simulink model "Sub3_2023"  (R2023b)
settings: Solver=FixedStepDiscrete  StartTime=0.0  StopTime=4.5  FixedStep=75e-6  RelTol=1e-3  EnableMultiTasking=on
undefined symbols (not defined in the file or in its folder): D1, D11, Delta
libraries: spsSeriesRLCBranchLib x41, spsLoadFlowBusLib x29, spsDistributedParametersLineLib x19, spsThreePhaseSeriesRLCLoadLib x15, spsThreePhaseTransformerTwoWindingsLib x13, spsThreePhaseParallelRLCLoadLib x11, spsThreePhaseVIMeasurementLib x11, spsSynchronousMachinepuStandardLib x7, spsExcitationSystemLib x7, spsHydraulicTurbineandGovernorLib x7, spsGenericPowerSystemStabilizerLib x7, spsMultiBandPowerSystemStabilizerLib x7
(part 3 of 5)

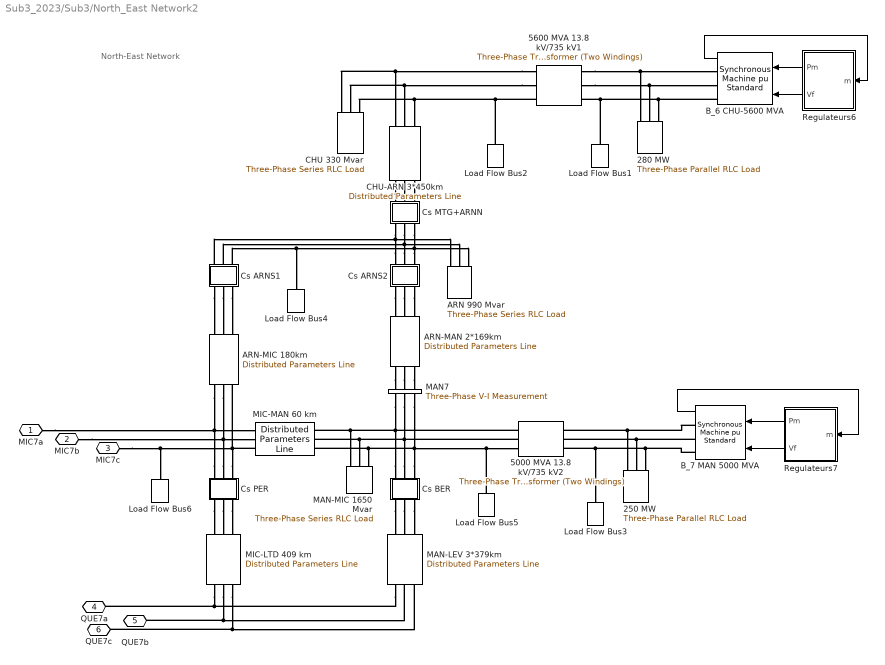
== system Sub3_2023/Sub3/North_East Network2 ==
  note: North-East Network
  250 MW : spsThreePhaseParallelRLCLoadLib/Three-Phase Parallel RLC Load  LConnTagsString=A|B|C  Configuration=Y (grounded)  NominalVoltage=(13800)*1  Vabc=[1e3 1e3 1e3]  Vabcp=[1e3 1e3 1e3]  NominalFrequency=60  UnbalancedPower=off  ActivePower=250000000  InductivePower=0  CapacitivePower=0  Pabc=[10e3 9e3 11e3]  QLabc=[100 90 110]  QCabc=[100 90 110]  Pabcp=[10e3 9e3 11e3]  QLabcp=[100 90 110]  QCabcp=[100 90 110]  Measurements=None  LoadType=constant PQ
  280 MW : spsThreePhaseParallelRLCLoadLib/Three-Phase Parallel RLC Load  LConnTagsString=A|B|C  Configuration=Y (grounded)  NominalVoltage=(13800)*1  Vabc=[1e3 1e3 1e3]  Vabcp=[1e3 1e3 1e3]  NominalFrequency=60  UnbalancedPower=off  ActivePower=280000000  InductivePower=0  CapacitivePower=0  Pabc=[10e3 9e3 11e3]  QLabc=[100 90 110]  QCabc=[100 90 110]  Pabcp=[10e3 9e3 11e3]  QLabcp=[100 90 110]  QCabcp=[100 90 110]  Measurements=None  LoadType=constant PQ
  5000 MVA 13.8 kV/735 kV2 : spsThreePhaseTransformerTwoWindingsLib/Three-Phase Transformer (Two Windings)  Winding1Connection=Delta (D1)  Winding2Connection=Yg  CoreType=Three single-phase transformers  SetSaturation=off  Hysteresis=off  DataFile='basic_model'  SetInitialFlux=off  Measurements=None  UNITS=pu  NominalPower=[ 5000e6 60 ]  Winding1="[ 13.8e3 0.002  0.0]"  Winding2=[ 735e3 0.002 0.12]  Rm=500  Lm=500  L0=0.5  Saturation="[ 0,0  ;  0.005,1.2  ;  1.0,1.4 ]"  InitialFluxes=[ 0.8 , -0.8 , 0.7 ]  BreakLoop=off  DiscreteSolver=Trapezoidal iterative  DataType=off  TransfoNumber=0
  5600 MVA 13.8 kV/735 kV1 : spsThreePhaseTransformerTwoWindingsLib/Three-Phase Transformer (Two Windings)  Winding1Connection=Delta (D1)  Winding2Connection=Yg  CoreType=Three single-phase transformers  SetSaturation=off  Hysteresis=off  DataFile='basic_model'  SetInitialFlux=off  Measurements=None  UNITS=pu  NominalPower=[ 5600e6 60 ]  Winding1="[ 13.8e3 0.002  0.0]"  Winding2=[ 735e3 0.002 0.12]  Rm=500  Lm=500  L0=0.5  Saturation="[ 0,0  ;  0.005,1.2  ;  1.0,1.4 ]"  InitialFluxes=[ 0.8 , -0.8 , 0.7 ]  BreakLoop=off  DiscreteSolver=Trapezoidal iterative  DataType=off  TransfoNumber=0
  ARN 990 Mvar : spsThreePhaseSeriesRLCLoadLib/Three-Phase Series RLC Load  LConnTagsString=A|B|C  Configuration=Y (grounded)  NominalVoltage=735e3  Vabc=[1e3 1e3 1e3]  Vabcp=[1e3 1e3 1e3]  NominalFrequency=60  UnbalancedPower=off  ActivePower=3300000  InductivePower=990e6  CapacitivePower=0  Pabc=[10e3 9e3 11e3]  QLabc=[100 90 110]  QCabc=[100 90 110]  Pabcp=[10e3 9e3 11e3]  QLabcp=[100 90 110]  QCabcp=[100 90 110]  Measurements=None  LoadType=constant Z
  ARN-MAN 2*169km : spsDistributedParametersLineLib/Distributed Parameters Line  Phases=3  Length=169  Frequency=60  Resistance="[0.01273  0.3864]/2"  Inductance="[0.9337e-3  4.1264e-3]/2"  Capacitance=[12.74e-9 7.751e-9]*2  x1=[-0.000975 1.67472397753016e-09 276427.2961151 -784420.047795512;-0.0009 1.60147333737436e-09 298492.841238193 -776291.834335293;-0.000825 1.52694250393602e-09 320319.775751095 -767543.06506037;-0.00075 1.45119105602304e-09 341890.651536318 -758180.733603041;-0.000675 1.37427954818385e-09 363188.225165806 -748212.324067824;-0.0006 1.29626946230102e-09 384195.471685062 -737645.805048779;-0.000525 1.21722315844361e-09 404895.598222641 -726489.623259537;-0.00045 1.13720382501748e-09 425272.057414111 -714752.696781126;-0.000375 1.05627542825344e-09 445308.560629765 -702444.407932991;-0.0003 9.74502661073603e-10 464989.090995501 -689574.595772914;-0.000225 8.91950891376898e-10 484297.916196467 -676153.548231822;-0.00015 8.08686109784932e-10 503219.601053231 -662191.993889769;-7.5e-05 7.24774876890116e-10 521739.019860433 -647701.093399678]  x2=[-0.000975 1.45072483719961e-09 170603.864508841 -782532.609847126;-0.0009 1.40774718437802e-09 192658.333570929 -777396.800423857;-0.000825 1.36364419999649e-09 214558.794508932 -771639.551892899;-0.00075 1.31845113930594e-09 236287.740429464 -765265.466510639;-0.000675 1.2722041289476e-09 257827.80154562 -758279.639623405;-0.0006 1.22494013807397e-09 279161.759062119 -750687.655594323;-0.000525 1.17669694879617e-09 300272.558939742 -742495.583339266;-0.00045 1.12751312598156e-09 321143.325528072 -733709.97147545;-0.000375 1.07742798642558e-09 341757.375055633 -724337.843086576;-0.0003 1.02648156742245e-09 362098.228966637 -714386.690108679;-0.000225 9.7471459476002e-10 382149.627093695 -703864.467341192;-0.00015 9.2216845016417e-10 401895.540655938 -692779.586088001;-7.5e-05 8.68885138218909e-10 421320.18507219 -681140.907433573]  x3=[-0.000975 -1.05058696200227e-12 1329.17201367209 -2414.87241463344;-0.0009 -1.27237442727808e-12 1396.90953145506 -2376.33167069217;-0.000825 -1.4931447759047e-12 1463.53038113202 -2335.89132357245;-0.00075 -1.71272152744335e-12 1528.98130701506 -2293.58370066899;-0.000675 -1.93092915559848e-12 1593.20998863548 -2249.44262204823;-0.0006 -2.14759322853083e-12 1656.16508256791 -2203.50337341303;-0.000525 -2.36254054829557e-12 1717.79626347352 -2155.80267789586;-0.00045 -2.57559928929408e-12 1778.05426432926 -2106.37866670286;-0.000375 -2.78659913562873e-12 1836.89091581125 -2055.27084863238;-0.0003 -2.99537141725075e-12 1894.2591848005 -2002.52007849219;-0.000225 -3.20174924479254e-12 1950.11321198057 -1948.16852444085;-0.00015 -3.40556764297644e-12 2004.40834849671 -1892.25963427904;-7.5e-05 -3.60666368249349e-12 2057.10119164754 -1834.83810071814]  x4=[-0.000975 1.05706410418254e-11 681.724417840617 -9455.17189861369;-0.0009 1.03719190093797e-11 948.756484621806 -9432.11979189245;-0.000825 1.01649058235736e-11 1215.03012998565 -9401.52779292584;-0.00075 9.94976696758033e-12 1480.33249885417 -9363.42035648977;-0.000675 9.72667442010975e-12 1744.45151257295 -9317.82794508585;-0.0006 9.49580651793084e-12 2007.17603844358 -9264.78700459018;-0.000525 9.25734781331221e-12 2268.2960584999 -9204.33993511903;-0.00045 9.01148892649379e-12 2527.60283739316 -9136.53505713488;-0.000375 8.75842639330793e-12 2784.88908925182 -9061.42657281972;-0.0003 8.49836250807169e-12 3039.94914338276 -8979.07452274673;-0.000225 8.23150516187579e-12 3292.57910868127 -8889.5447378847;-0.00015 7.95806767639975e-12 3542.57703661844 -8792.9087869738;-7.5e-05 7.67826863338571e-12 3789.74308267579 -8689.24391931461]  x5=0.000955765248222805  V1=ones(3,3)  V2=ones(3,3)  I1=ones(3,3)  I2=ones(3,3)  nHarmo=1  Measurements=None  Decoupling=on  VsMag0=[679080.965035231 679082.342856258 679080.506296754]  VrMag0=[653943.402704874 653944.061381525 653943.21471976]  VsAngle0=[10.4723030523858 -109.527808757282 130.47214647176]  VrAngle0=[3.35889302260881 -116.641159315006 123.358816875026]  IsMag0=[2259.59659727673 2259.62910082009 2259.62302792986]  IrMag0=[7771.0084515065 7771.00049259901 7770.97273571619]  IsAngle0=[19.8888438810525 -100.110858095203 139.888279140942]  IrAngle0=[-4.81594167232723 -124.81621186364 115.183974051697]
      settings: AttributesFormatString=\n  LibrarySourceBlock=sps_lib/Power Grid Elements/Distributed Parameters Line
  ARN-MIC 180km : spsDistributedParametersLineLib/Distributed Parameters Line  Phases=3  Length=180  Frequency=60  Resistance="[0.01273  0.3864]"  Inductance="[0.9337e-3  4.1264e-3]"  Capacitance=[12.74e-9 7.751e-9]  x1=[-0.00105 1.24724783260845e-09 262529.955827382 -774207.772445515;-0.000975 1.17944476350714e-09 284312.349574646 -766476.523484134;-0.0009 1.110698864308e-09 305867.468379784 -758132.564917363;-0.000825 1.04106508943099e-09 327178.081410629 -749182.566778015;-0.00075 9.70599103050325e-10 348227.153289186 -739633.683557663;-0.000675 8.99357234597342e-10 368997.857709458 -729493.548487449;-0.0006 8.27396433731648e-10 389473.590888134 -718770.2674362;-0.000525 7.5477422481642e-10 409637.9848374 -707472.412430716;-0.00045 6.81548660934306e-10 429474.920449258 -695609.014803426;-0.000375 6.07778277480686e-10 448968.540380895 -683189.557972877;-0.0003 5.33522045371367e-10 468103.261730801 -670223.969862836;-0.000225 4.58839323902139e-10 486863.7884955 -656722.614966056;-0.00015 3.83789813297861e-10 505235.12379694 -642696.286059066;-7.5e-05 3.08433506989013e-10 523202.581870775 -628156.195574583]  x2=[-0.00105 4.58025582629427e-09 126759.491965629 -811882.989724212;-0.000975 4.52463715432621e-09 149661.239004177 -807974.954382897;-0.0009 4.46540155664625e-09 172443.34913816 -803421.036225481;-0.000825 4.40259638528484e-09 195087.610697313 -798224.87558446;-0.00075 4.33627184573503e-09 217575.922205416 -792390.626191147;-0.000675 4.26648095681891e-09 239890.30685033 -785922.95185524;-0.0006 4.19327950830526e-09 262012.926854394 -778827.022736644;-0.000525 4.116726016312e-09 283926.097733662 -771108.511212526;-0.00045 4.03688167652932e-09 305612.302434616 -762773.5873429;-0.000375 3.95381031530078e-09 327054.20533703 -753828.913938379;-0.0003 3.86757833860152e-09 348234.666111794 -744281.641234026;-0.000225 3.77825467895431e-09 369136.753422638 -734139.401173561;-0.00015 3.68591074032598e-09 389743.758460777 -723410.301308507;-7.5e-05 3.59062034104816e-09 410039.208301682 -712102.918317136]  x3=[-0.00105 2.96537177276768e-12 -44.8517351582774 -825.879343626536;-0.000975 3.21260661019266e-12 -21.4861584035534 -826.817643960417;-0.0009 3.45727333904798e-12 1.89659405744908 -827.094998920449;-0.000825 3.69917637649412e-12 25.2778304101809 -826.711186793323;-0.00075 3.93812234894418e-12 48.6388600520466 -825.66651439258;-0.000675 4.17392024664379e-12 71.9610085333863 -823.961816813352;-0.0006 4.40638157636136e-12 95.2256324855447 -821.598456764802;-0.000525 4.63532051206668e-12 118.414134524095 -818.578323480792;-0.00045 4.86055404347744e-12 141.507978115304 -814.90383120966;-0.000375 5.08190212235481e-12 164.488702393952 -810.577917284306;-0.0003 5.29918780643128e-12 187.337936920669 -805.604039774133;-0.000225 5.51223740085559e-12 210.037416366977 -799.98617472072;-0.00015 5.7208805970417e-12 232.568995116322 -793.728812959434;-7.5e-05 5.92495060881096e-12 254.914661769395 -786.836956529526]  x4=[-0.00105 4.18543085449922e-12 787.856966725132 -5164.02437043793;-0.000975 3.74166953826904e-12 933.532622338205 -5139.68710729476;-0.0009 3.29491718865944e-12 1078.46202625651 -5111.24125691787;-0.000825 2.84553093266314e-12 1222.52932413205 -5078.7095584848;-0.00075 2.39387000277736e-12 1365.6193507712 -5042.11801733755;-0.000675 1.94029544983879e-12 1507.61772219602 -5001.49588419424;-0.0006 1.48516985440514e-12 1648.41092708104 -4956.87563176655;-0.000525 1.02885703691374e-12 1787.88641749249 -4908.29292880156;-0.00045 5.71721766849072e-13 1925.93269885737 -4855.78661156869;-0.000375 1.1412947115162e-13 2062.43941909055 -4799.39865281457;-0.0003 -3.43554057898831e-13 2197.29745680848 -4739.17412821064;-0.000225 -8.00962955091952e-13 2330.39900855922 -4675.16118032042;-0.00015 -1.25773157475392e-12 2461.63767499882 -4607.41098011501;-7.5e-05 -1.71349478303896e-12 2590.90854594535 -4535.97768606785]  x5=0.00101797482059234  V1=ones(3,3)  V2=ones(3,3)  I1=ones(3,3)  I2=ones(3,3)  nHarmo=1  Measurements=None  Decoupling=on  VsMag0=[667492.500318924 667493.817536521 667492.030186015]  VrMag0=[670930.718084371 670931.402748966 670930.538861449]  VsAngle0=[11.411536339946 -108.588575536847 131.411382483005]  VrAngle0=[1.55396261636306 -118.446088813405 121.553886266144]  IsMag0=[678.171382863083 678.181184846405 678.186053011925]  IrMag0=[4283.30300695141 4283.29854095568 4283.28683546869]  IsAngle0=[-10.4293295371495 -130.428376510203 109.570429815951]  IrAngle0=[1.35460954054908 -118.645605751909 121.354553630563]
      settings: AttributesFormatString=\n  LibrarySourceBlock=sps_lib/Power Grid Elements/Distributed Parameters Line
  "B_6 CHU-5600 MVA " : spsSynchronousMachinepuStandardLib/Synchronous Machine pu Standard  PresetModel=No  MechanicalLoad=Mechanical power Pm  ShowDetailedParameters=on  RotorType=Salient-pole  Units=per unit standard parameters  MeasurementBus=off  NominalParameters="[ 5600E6  13800   60 ]"  Reactances1=[ 31 32 33 34 35 36 37 ]  Reactances2=[ 1.305, 0.296, 0.252, 0.474, 0.243, 0.18 ]  dAxisTimeConstants=Short-circuit  qAxisTimeConstants=Open-circuit  TimeConstants1=[]  TimeConstants2=[]  TimeConstants3=[]  TimeConstants4=[]  TimeConstants5=[ 1.01, 0.053, 0.1 ]  TimeConstants6=[]  TimeConstants7=[]  TimeConstants8=[]  StatorResistance=2.8544e-3  Mechanical="[ 4.0 0  32]"  PolePairs=32  InitialConditions=[0 -61.7964 0.894782 0.894782 0.894782 8.48442 -111.516 128.484 1.31361]  SetSaturation=off  Saturation=[0.6404,0.7127,0.8441,0.9214,0.9956,1.082,1.19,1.316,1.457;0.7,0.7698,0.8872,0.9466,0.9969,1.046,1.1,1.151,1.201]  LoadFlowParameters=[1 5000000000 0 0 0]  TsPowergui=0  TsBlock=-1  IterativeModel=Trapezoidal non iterative  IterativeDiscreteModel=Trapezoidal non iterative  BusType=PV  Pref=5000000000  Qref=0  Qmin=-Inf  Qmax=Inf  PLF=0  QLF=0
  B_7 MAN 5000 MVA : spsSynchronousMachinepuStandardLib/Synchronous Machine pu Standard  PresetModel=No  MechanicalLoad=Mechanical power Pm  ShowDetailedParameters=on  RotorType=Salient-pole  Units=per unit standard parameters  MeasurementBus=off  NominalParameters="[ 5000E6  13800   60 ]"  Reactances1=[ 31 32 33 34 35 36 37 ]  Reactances2=[ 1.305, 0.296, 0.252, 0.474, 0.243, 0.18 ]  dAxisTimeConstants=Short-circuit  qAxisTimeConstants=Open-circuit  TimeConstants1=[]  TimeConstants2=[]  TimeConstants3=[]  TimeConstants4=[]  TimeConstants5=[ 1.01, 0.053, 0.1 ]  TimeConstants6=[]  TimeConstants7=[]  TimeConstants8=[]  StatorResistance=2.8544e-3  Mechanical="[ 3.7 0  32]"  PolePairs=32  InitialConditions=[0 -81.9543 0.907703 0.907703 0.907703 -8.76021 -128.76 111.24 1.25655]  SetSaturation=off  Saturation=[0.6404,0.7127,0.8441,0.9214,0.9956,1.082,1.19,1.316,1.457;0.7,0.7698,0.8872,0.9466,0.9969,1.046,1.1,1.151,1.201]  LoadFlowParameters=[1 4500000000 0 0 0]  TsPowergui=0  TsBlock=-1  IterativeModel=Trapezoidal non iterative  IterativeDiscreteModel=Trapezoidal non iterative  BusType=PV  Pref=4500000000  Qref=0  Qmin=-Inf  Qmax=Inf  PLF=0  QLF=0
  CHU 330 Mvar : spsThreePhaseSeriesRLCLoadLib/Three-Phase Series RLC Load  LConnTagsString=A|B|C  Configuration=Y (grounded)  NominalVoltage=735e3  Vabc=[1e3 1e3 1e3]  Vabcp=[1e3 1e3 1e3]  NominalFrequency=60  UnbalancedPower=off  ActivePower=1100000  InductivePower=330e6  CapacitivePower=0  Pabc=[10e3 9e3 11e3]  QLabc=[100 90 110]  QCabc=[100 90 110]  Pabcp=[10e3 9e3 11e3]  QLabcp=[100 90 110]  QCabcp=[100 90 110]  Measurements=None  LoadType=constant Z
  CHU-ARN 3*450km : spsDistributedParametersLineLib/Distributed Parameters Line  Phases=3  Length=450  Frequency=60  Resistance="[0.01273  0.3864]/3"  Inductance="[0.9337e-3  4.1264e-3]/3"  Capacitance=[12.74e-9 7.751e-9]*3  x1=[-0.00255 1.77535384487348e-09 0 0;-0.002475 1.68842898528115e-09 0 0;-0.0024 1.60015442139181e-09 0 0;-0.002325 1.5106007185412e-09 0 0;-0.00225 1.41983946458915e-09 0 0;-0.002175 1.32794321269338e-09 0 0;-0.0021 1.23498542331159e-09 0 0;-0.002025 1.14104040547832e-09 0 0;-0.00195 1.04618325740342e-09 0 0;-0.001875 9.50489806439687e-10 0 0;-0.0018 8.54036548467669e-10 0 0;-0.001725 7.56900586746003e-10 0 0;-0.00165 6.59159570276259e-10 0 0;-0.001575 5.60891631731516e-10 242668.421457002 -732167.508894334;-0.0015 4.62175324998297e-10 263270.288908672 -725014.59046711;-0.001425 3.63089562381793e-10 283661.702119559 -717282.106469362;-0.00135 2.63713551524579e-10 303826.360505941 -708976.238130487;-0.001275 1.64126732089228e-10 323748.144748434 -700103.62503455;-0.0012 6.44087122554682e-11 343411.129677528 -690671.359812705;-0.001125 -3.53607949173821e-11 362799.597003924 -680686.982473452;-0.00105 -1.35102035211814e-10 381898.047883495 -670158.47437527;-0.000975 -2.34735277006428e-10 400691.215306824 -659094.251846441;-0.0009 -3.34180875012173e-10 419164.076303418 -647503.159457166;-0.000825 -4.33359333939572e-10 437301.86395084 -635394.462949351;-0.00075 -5.3219137204604e-10 455090.079179163 -622777.841829716;-0.000675 -6.30597984512496e-10 472514.502361302 -609663.381632143;-0.0006 -7.28500506598605e-10 489561.204679968 -596061.565855456;-0.000525 -8.2582067652617e-10 506216.55926215 -581983.267583072;-0.00045 -9.22480698040401e-10 522467.252072231 -567439.740791224;-0.000375 -1.01840330259905e-09 538300.292555022 -552442.611352707;-0.0003 -1.11351181113969e-09 553703.024020216 -537003.86774333;-0.000225 -1.2077301953758e-09 568663.133759948 -521135.851458514;-0.00015 -1.30098313857263e-09 583168.66289139 -504851.247147688;-7.5e-05 -1.39319609575419e-09 597208.015916497 -488163.072474375]  x2=[-0.00255 2.72407888436873e-09 0 0;-0.002475 2.6953160484316e-09 0 0;-0.0024 2.66439861808508e-09 0 0;-0.002325 2.63135130824993e-09 0 0;-0.00225 2.59620053643998e-09 0 0;-0.002175 2.55897440164441e-09 0 0;-0.0021 2.51970266186578e-09 0 0;-0.002025 2.478416710332e-09 0 0;-0.00195 2.43514955040103e-09 0 0;-0.001875 2.38993576917851e-09 0 0;-0.0018 2.34281150986935e-09 0 0;-0.001725 2.29381444288541e-09 0 0;-0.00165 2.24298373573238e-09 0 0;-0.001575 2.1903600216998e-09 -54170.2857367538 -807523.190587141;-0.0015 2.1359853673795e-09 -31319.4766466804 -808731.868853748;-0.001425 2.0799032390382e-09 -8443.63124617975 -809294.059238405;-0.00135 2.02215846787119e-09 14438.9638639472 -809209.312334721;-0.001275 1.96279721416503e-09 37310.0166872849 -808477.695888074;-0.0012 1.90186693039767e-09 60151.2444541452 -807099.794741458;-0.001125 1.83941632330569e-09 82944.3882365337 -805076.710367967;-0.00105 1.77549531494887e-09 105671.227544058 -802410.059990295;-0.000975 1.71015500280328e-09 128313.594889107 -799101.975287951;-0.0009 1.64344761891469e-09 150853.390309666 -795155.100693233;-0.000825 1.57542648814513e-09 173272.595838145 -790572.591277302;-0.00075 1.50614598554578e-09 195553.289904671 -785358.110228069;-0.000675 1.43566149289039e-09 217677.661663313 -779515.825921903;-0.0006 1.36402935440395e-09 239628.025229801 -773050.408591487;-0.000525 1.29130683172194e-09 261386.833819352 -765967.02659251;-0.00045 1.21755205811631e-09 282936.693773301 -758271.342272164;-0.000375 1.1428239920246e-09 304260.378463324 -749969.507442746;-0.0003 1.06718236991945e-09 325340.842062143 -741068.158463997;-0.000225 9.90687658556226e-10 346161.2331697 -731574.410938095;-0.00015 9.13401006636783e-10 366704.908283905 -721495.854021552;-7.5e-05 8.35384195928139e-10 386955.445105201 -710840.544358562]  x3=[-0.00255 5.00391490531751e-12 0 0;-0.002475 4.937944497013e-12 0 0;-0.0024 4.86802677143067e-12 0 0;-0.002325 4.79421761973056e-12 0 0;-0.00225 4.71657604381923e-12 0 0;-0.002175 4.6351641091845e-12 0 0;-0.0021 4.55004689528128e-12 0 0;-0.002025 4.46129244350803e-12 0 0;-0.00195 4.36897170281549e-12 0 0;-0.001875 4.27315847299124e-12 0 0;-0.0018 4.17392934566519e-12 0 0;-0.001725 4.07136364308348e-12 0 0;-0.00165 3.96554335469944e-12 0 0;-0.001575 3.8565530716325e-12 -1464.09976005058 -2947.40439174839;-0.0015 3.74447991904734e-12 -1380.19037065337 -2987.6190390229;-0.001425 3.62941348650736e-12 -1295.17767819147 -3025.44542934972;-0.00135 3.51144575635815e-12 -1209.12964051052 -3060.85332489118;-0.001275 3.39067103019823e-12 -1122.11504309524 -3093.81442111735;-0.0012 3.26718585349578e-12 -1034.20344408345 -3124.30236943223;-0.001125 3.14108893841166e-12 -945.465118662299 -3152.29279823642;-0.00105 3.01248108489045e-12 -855.971002891393 -3177.76333240939;-0.000975 2.88146510008248e-12 -765.792636997571 -3200.69361119584;-0.0009 2.7481457161614e-12 -675.002108186754 -3221.06530448176;-0.000825 2.61262950660287e-12 -583.671993018531 -3238.86212744722;-0.00075 2.47502480099132e-12 -491.875299389569 -3254.06985358426;-0.000675 2.33544159842301e-12 -399.68540817222 -3266.67632606928;-0.0006 2.19399147957438e-12 -307.176014554971 -3276.67146748106;-0.000525 2.05078751750617e-12 -214.421069131637 -3284.0472878565;-0.00045 1.90594418727457e-12 -121.49471878639 -3288.79789107763;-0.000375 1.75957727442158e-12 -28.4712474218783 -3290.91947958492;-0.0003 1.61180378241786e-12 64.5749834221983 -3290.410357413;-0.000225 1.4627418391319e-12 157.569594012558 -3287.27093154632;-0.00015 1.31251060240043e-12 250.438245880359 -3281.5037115939;-7.5e-05 1.1612301647755e-12 343.106701246237 -3273.11330778312]  x4=[-0.00255 2.07056787924814e-11 0 0;-0.002475 2.05392287535775e-11 0 0;-0.0024 2.03563599694686e-11 0 0;-0.002325 2.0157218622663e-11 0 0;-0.00225 1.99419639037061e-11 0 0;-0.002175 1.97107678839269e-11 0 0;-0.0021 1.94638153778862e-11 0 0;-0.002025 1.92013037956387e-11 0 0;-0.00195 1.89234429849269e-11 0 0;-0.001875 1.86304550634312e-11 0 0;-0.0018 1.83225742412134e-11 0 0;-0.001725 1.80000466334919e-11 0 0;-0.00165 1.76631300639015e-11 0 0;-0.001575 1.73120938583931e-11 -1565.83540459126 -14460.8260986628;-0.0015 1.69472186299381e-11 -1156.39187005824 -14499.3124213109;-0.001425 1.65687960542115e-11 -746.023933557683 -14526.2082154564;-0.00135 1.61771286364303e-11 -335.059636939191 -14541.4919810129;-0.001275 1.57725294695355e-11 76.1725012264878 -14545.1515003721;-0.0012 1.53553219839105e-11 487.343748260165 -14537.1838481701;-0.001125 1.49258396888359e-11 898.12542015809 -14517.5953936263;-0.00105 1.4484425905887e-11 1308.18914433692 -14486.4017954515;-0.000975 1.40314334944881e-11 1717.20712212974 -14443.6279893308;-0.0009 1.35672245698418e-11 2124.85239082327 -14389.3081679903;-0.000825 1.309217021346e-11 2530.79908502691 -14323.4857538641;-0.00075 1.26066501765264e-11 2934.72269716451 -14246.213364383;-0.000675 1.21110525763298e-11 3336.30033688075 -14157.5527699127;-0.0006 1.16057735860091e-11 3735.2109891548 -14057.5748443761;-0.000525 1.10912171178581e-11 4131.13577091476 -13946.3595085969;-0.00045 1.05677945004443e-11 4523.75818594796 -13823.995666413;-0.000375 1.00359241497996e-11 4912.76437790312 -13690.5811336076;-0.0003 9.49603123494424e-12 5297.84338118241 -13546.2225597169;-0.000225 8.94854733801387e-12 5678.6873695225 -13391.0353427762;-0.00015 8.39391010925885e-12 6054.99190206622 -13225.1435370721;-7.5e-05 7.83256291719362e-12 6426.45616672792 -13048.679753976]  x5=0.00254493705148084  V1=ones(3,3)  V2=ones(3,3)  I1=ones(3,3)  I2=ones(3,3)  nHarmo=1  Measurements=None  Decoupling=on  VsMag0=[629792.481623588 629794.239253248 629791.265031449]  VrMag0=[660822.002060051 660822.3945477 660821.800733033]  VsAngle0=[22.3571846561361 -97.6430354653559 142.35693611621]  VrAngle0=[0.182246528177579 -119.817793275386 120.182197155388]  IsMag0=[2715.66118101541 2715.69463660348 2715.7067900314]  IrMag0=[12002.6021032757 12002.5859963177 12002.5499905583]  IsAngle0=[-22.3962421231226 -142.395538520012 97.6034984021941]  IrAngle0=[-2.15980439261933 -122.160047251329 117.840140765692]
      settings: AttributesFormatString=\n  LibrarySourceBlock=sps_lib/Power Grid Elements/Distributed Parameters Line
  "Cs ARNS1 " : Subsystem  mask{Xc=25}
      mask prompts: Xc "Condensator Reactance at  60Hz  (ohm):"
      mask help: Series Compensation
      mask init:
      | Cs=1/Xc/(2*pi*60);
      mask Display: disp('Cs')
  Cs ARNS2 : Subsystem  mask{Xc=25/2}
      mask prompts: Xc "Condensator Reactance at  60Hz  (ohm):"
      mask help: Series Compensation
      mask init:
      | Cs=1/Xc/(2*pi*60);
      mask Display: disp('Cs')
  Cs BER : Subsystem  mask{Xc=22/3}
      mask prompts: Xc "Condensator Reactance at  60Hz  (ohm):"
      mask help: Series Compensation
      mask init:
      | Cs=1/Xc/(2*pi*60);
      mask Display: disp('Cs')
  "Cs MTG+ARNN " : Subsystem  mask{Xc=(30+25)/3}
      mask prompts: Xc "Condensator Reactance at  60Hz  (ohm):"
      mask help: Series Compensation
      mask init:
      | Cs=1/Xc/(2*pi*60);
      mask Display: disp('Cs')
  "Cs PER " : Subsystem  mask{Xc=22}
      mask prompts: Xc "Condensator Reactance at  60Hz  (ohm):"
      mask help: Series Compensation
      mask init:
      | Cs=1/Xc/(2*pi*60);
      mask Display: disp('Cs')
  Load Flow Bus1 : spsLoadFlowBusLib/Load Flow Bus  LConnTagsString=a  Phases=single  Connectors=on one side  ID=CHU_13.8  Vbase=13.8e3  Vref=1  Vangle=0  VLF=1  VLFb=1  VLFc=1  angleLF=4.726  angleLFb=0  angleLFc=0
      settings: AttributesFormatString=%<ID>\n%<Vbase>V\n%<VLF>pu\n%<angleLF>deg.
  Load Flow Bus2 : spsLoadFlowBusLib/Load Flow Bus  LConnTagsString=a  Phases=single  Connectors=on one side  ID=CHU7  Vbase=735e3  Vref=1  Vangle=0  VLF=1.009  VLFb=1  VLFc=1  angleLF=28.97  angleLFb=0  angleLFc=0
      settings: AttributesFormatString=%<ID>\n%<Vbase>V\n%<VLF>pu\n%<angleLF>deg.
  Load Flow Bus3 : spsLoadFlowBusLib/Load Flow Bus  LConnTagsString=a  Phases=single  Connectors=on one side  ID=MAN_13.8  Vbase=13.8e3  Vref=1  Vangle=0  VLF=1  VLFb=1  VLFc=1  angleLF=-16.23  angleLFb=0  angleLFc=0
      settings: AttributesFormatString=%<ID>\n%<Vbase>V\n%<VLF>pu\n%<angleLF>deg.
  Load Flow Bus4 : spsLoadFlowBusLib/Load Flow Bus  LConnTagsString=a  Phases=single  Connectors=on one side  ID=ARN7  Vbase=735e3  Vref=1  Vangle=0  VLF=1.054  VLFb=1  VLFc=1  angleLF=12.72  angleLFb=0  angleLFc=0
      settings: AttributesFormatString=%<ID>\n%<Vbase>V\n%<VLF>pu\n%<angleLF>deg.
  Load Flow Bus5 : spsLoadFlowBusLib/Load Flow Bus  LConnTagsString=a  Phases=single  Connectors=on one side  ID=MAN7  Vbase=735e3  Vref=1  Vangle=0  VLF=1.016  VLFb=1  VLFc=1  angleLF=7.996  angleLFb=0  angleLFc=0
      settings: AttributesFormatString=%<ID>\n%<Vbase>V\n%<VLF>pu\n%<angleLF>deg.
  Load Flow Bus6 : spsLoadFlowBusLib/Load Flow Bus  LConnTagsString=a  Phases=single  Connectors=on one side  ID=MIC7  Vbase=735e3  Vref=1  Vangle=0  VLF=1.041  VLFb=1  VLFc=1  angleLF=5.981  angleLFb=0  angleLFc=0
      settings: AttributesFormatString=%<ID>\n%<Vbase>V\n%<VLF>pu\n%<angleLF>deg.
  MAN-LEV 3*379km : spsDistributedParametersLineLib/Distributed Parameters Line  Phases=3  Length=379  Frequency=60  Resistance="[0.01273  0.3864]/3"  Inductance="[0.9337e-3  4.1264e-3]/3"  Capacitance=[12.74e-9 7.751e-9]*3  x1=[-0.002175 3.19869160212258e-09 -129715.856576142 -778750.814672859;-0.0021 3.15804297327423e-09 -107648.251269302 -782106.718665368;-0.002025 3.11486985319272e-09 -85494.5935974704 -784837.41851361;-0.00195 3.06920675380967e-09 -63272.5928556284 -786940.731337907;-0.001875 3.02109017750807e-09 -41000.0129711608 -788414.975782169;-0.0018 2.9705585879428e-09 -18694.6583036453 -789258.973357945;-0.001725 2.9176523792934e-09 3625.64058768033 -789472.049386487;-0.00165 2.86241384397356e-09 25943.0411973943 -789054.033538075;-0.001575 2.80488713882326e-09 48239.703336917 -788005.259968185;-0.0015 2.74511824981039e-09 70497.8033956842 -786326.567050362;-0.001425 2.68315495527035e-09 92699.5485890696 -784019.296706038;-0.00135 2.6190467877127e-09 114827.191181663 -781085.293331825;-0.001275 2.55284499422572e-09 136863.042674542 -777526.902325128;-0.0012 2.4846024955102e-09 158789.487945181 -773346.968209273;-0.001125 2.41437384357545e-09 180588.999328717 -768548.832359637;-0.00105 2.34221517813131e-09 202244.150629294 -763136.330332604;-0.000975 2.26818418171087e-09 223737.631050298 -757113.78879948;-0.0009 2.19234003355995e-09 245052.25903234 -750486.02208782;-0.000825 2.11474336233012e-09 266170.995987937 -743258.328332924;-0.00075 2.03545619761311e-09 287076.959921894 -735436.485242592;-0.000675 1.95454192035525e-09 307753.438926515 -727026.745478513;-0.0006 1.87206521219176e-09 328183.904540843 -718035.83165798;-0.000525 1.78809200374119e-09 348352.024963263 -708470.930979937;-0.00045 1.70268942190156e-09 368241.678106893 -698339.689479638;-0.000375 1.61592573619009e-09 387836.96448733 -687650.205916523;-0.0003 1.52787030416959e-09 407122.219932461 -676411.0253002;-0.000225 1.43859351600514e-09 426082.028104156 -664631.132059688;-0.00015 1.34816673819522e-09 444701.232821859 -652319.942861405;-7.5e-05 1.25666225652243e-09 462964.950178201 -639487.299081628]  x2=[-0.002175 1.41720579426248e-08 -453830.168532079 -672756.853007256;-0.0021 1.4238167680244e-08 -434629.546160119 -685317.991887117;-0.002025 1.42928956444709e-08 -415081.487579013 -697331.298049981;-0.00195 1.43361980866081e-08 -395201.619207697 -708787.16824271;-0.001875 1.43680403913462e-08 -375005.832708773 -719676.444817953;-0.0018 1.43883971044338e-08 -354510.272284963 -729990.423054628;-0.001725 1.4397251953026e-08 -333731.321773678 -739720.85811634;-0.00165 1.43945978586922e-08 -312685.591550028 -748859.971642184;-0.001575 1.4380436943075e-08 -291389.905248742 -757400.457964638;-0.0015 1.43547805261935e-08 -269861.286315616 -765335.489949611;-0.001425 1.43176491173949e-08 -248116.944399225 -772658.724453944;-0.00135 1.42690723989592e-08 -226174.261593798 -779364.307396023;-0.001275 1.4209089202372e-08 -204050.778544234 -785446.878435444;-0.0012 1.41377474772827e-08 -181764.180424385 -790901.575257983;-0.001125 1.40551042531748e-08 -159332.282799789 -795724.037462462;-0.00105 1.39612255937773e-08 -136773.017386189 -799910.410046378;-0.000975 1.3856186544254e-08 -114104.417715188 -803457.346487544;-0.0009 1.3740071071214e-08 -91344.604718521 -806362.011419237;-0.000825 1.36129719955899e-08 -68511.7722424616 -808622.082896754;-0.00075 1.34749909184379e-08 -45624.1725039369 -810235.754253535;-0.000675 1.33262381397199e-08 -22700.1014999858 -811201.73554539;-0.0006 1.31668325701314e-08 242.115617781237 -811519.254581652;-0.000525 1.29969016360456e-08 23184.1391920279 -811188.057542463;-0.00045 1.28165811776512e-08 46107.6297201337 -810208.409181668;-0.000375 1.26260153403637e-08 68994.2625145116 -808581.092615177;-0.0003 1.24253564595976e-08 91825.742351083 -806307.408694955;-0.000225 1.2214764938992e-08 114583.8180942 -803389.17496914;-0.00015 1.19944091221863e-08 137250.297286324 -799828.72422912;-7.5e-05 1.1764465158249e-08 159807.060690796 -795628.902644742]  x3=[-0.002175 4.30582667042764e-12 -1369.21748804157 -554.792265212319;-0.0021 5.94389643124348e-12 -1352.98611910174 -593.279680633568;-0.002025 7.57721473219686e-12 -1335.67319375967 -631.292837355603;-0.00195 9.2044759236286e-12 -1317.29255170301 -668.80134824256;-0.001875 1.08243791978402e-11 -1297.85888613576 -705.775229564736;-0.0018 1.24356296289396e-11 -1277.38773203284 -742.18492496712;-0.001725 1.40369392079851e-11 -1255.89545372162 -778.001329096296;-0.00165 1.56270278726001e-11 -1233.39923180054 -813.195810866812;-0.001575 1.72046245302354e-11 -1209.91704940521 -847.740236348435;-0.0015 1.87684680742607e-11 -1185.46767783293 -881.606991255981;-0.001425 2.03173083920747e-11 -1160.07066153725 -914.769003023756;-0.00135 2.18499073644253e-11 -1133.74630250442 -947.199762446949;-0.001275 2.33650398551435e-11 -1106.51564402426 -978.873344872684;-0.0012 2.48614946904987e-11 -1078.40045386853 -1009.76443092379;-0.001125 2.63380756273919e-11 -1049.42320689006 -1039.84832673873;-0.00105 2.77936023096146e-11 -1019.60706705671 -1069.1009837115;-0.000975 2.92269112114074e-11 -988.975868934467 -1097.49901771567;-0.0009 3.06368565675645e-11 -957.554098634438 -1125.01972779738;-0.000825 3.20223112893412e-11 -925.366874239029 -1151.64111432207;-0.00075 3.33821678654309e-11 -892.439925722941 -1177.34189656067;-0.000675 3.47153392472933e-11 -858.799574385019 -1202.10152970109;-0.0006 3.6020759718124e-11 -824.472711807408 -1225.90022127144;-0.000525 3.7297385744772e-11 -789.486778358834 -1248.71894696181;-0.00045 3.85441968119249e-11 -753.869741259192 -1270.53946583202;-0.000375 3.97601962378922e-11 -717.650072222982 -1291.34433489315;-0.0003 4.09444119713384e-11 -680.856724699451 -1311.11692305119;-0.000225 4.20958973683252e-11 -643.519110727652 -1329.84142440171;-0.00015 4.32137319490446e-11 -605.66707742491 -1347.50287086482;-7.5e-05 4.42970221336363e-11 -567.330883127492 -1364.08714415045]  x4=[-0.002175 5.52368172662519e-11 -9019.35016941144 -13700.3757737253;-0.0021 5.44254824531843e-11 -8628.42708034827 -13949.881495902;-0.002025 5.35706407421815e-11 -8230.60655869642 -14188.2358962513;-0.00195 5.26729754806276e-11 -7826.20661609405 -14415.2484379123;-0.001875 5.1733204248398e-11 -7415.55052366776 -14630.7376505328;-0.0018 5.07520782842369e-11 -6998.96655361457 -14834.5312753332;-0.001725 4.97303818852282e-11 -6576.7877167862 -15026.4664028081;-0.00165 4.86689317798407e-11 -6149.35149648526 -15206.3896029533;-0.001575 4.75685764750481e-11 -5716.99957868626 -15374.1570479153;-0.0015 4.6430195578045e-11 -5280.0775788971 -15529.6346269658;-0.001425 4.52546990931026e-11 -4838.93476587925 -15672.6980537069;-0.00135 4.40430266941253e-11 -4393.92378244774 -15803.2329654241;-0.001275 4.27961469734896e-11 -3945.40036357384 -15921.1350145064;-0.0012 4.15150566677663e-11 -3493.72305201594 -16026.3099518596;-0.001125 4.02007798609445e-11 -3039.25291170602 -16118.673702248;-0.00105 3.88543671657944e-11 -2582.3532391206 -16198.1524315029;-0.000975 3.74768948840237e-11 -2123.38927286717 -16264.682605544;-0.0009 3.60694641458984e-11 -1662.72790171795 -16318.2110411683;-0.000825 3.46332000300162e-11 -1200.73737132468 -16358.6949485632;-0.00075 3.31692506639357e-11 -737.786989848682 -16386.1019655127;-0.000675 3.16787863063811e-11 -274.246832741513 -16400.4101832667;-0.0006 3.01629984117548e-11 189.512553087631 -16401.608164055;-0.000525 2.86230986777075e-11 653.120445481477 -16389.6949502299;-0.00045 2.70603180765254e-11 1116.20624338428 -16364.6800650323;-0.000375 2.54759058711096e-11 1578.39976309465 -16326.5835049787;-0.0003 2.38711286163349e-11 2039.33153418474 -16275.4357238764;-0.000225 2.22472691465848e-11 2498.63309484921 -16211.2776084789;-0.00015 2.06056255502735e-11 2955.93728644803 -16134.1604458021;-7.5e-05 1.8947510132174e-11 3410.87854700741 -16044.1458821258]  x5=0.00214340253891386  V1=ones(3,3)  V2=ones(3,3)  I1=ones(3,3)  I2=ones(3,3)  nHarmo=1  Measurements=None  Decoupling=on  VsMag0=[644608.259457103 644608.981755965 644608.02280338]  VrMag0=[662602.894278608 662603.037872478 662602.726163221]  VsAngle0=[7.52314012710744 -112.476921228499 127.523053849326]  VrAngle0=[-17.0228975012821 -137.022921456009 102.977079768198]  IsMag0=[1217.04656467753 1217.04790828061 1217.06108392333]  IrMag0=[13512.6448948102 13512.6449098298 13512.625660389]  IsAngle0=[-50.9633701968684 -170.962617439536 69.036951403284]  IrAngle0=[-16.3779589453586 -136.378053156049 103.621993894143]
      settings: AttributesFormatString=\n  LibrarySourceBlock=sps_lib/Power Grid Elements/Distributed Parameters Line
  MAN-MIC 1650 Mvar : spsThreePhaseSeriesRLCLoadLib/Three-Phase Series RLC Load  LConnTagsString=A|B|C  Configuration=Y (grounded)  NominalVoltage=735e3  Vabc=[1e3 1e3 1e3]  Vabcp=[1e3 1e3 1e3]  NominalFrequency=60  UnbalancedPower=off  ActivePower=5500000  InductivePower=1650e6  CapacitivePower=0  Pabc=[10e3 9e3 11e3]  QLabc=[100 90 110]  QCabc=[100 90 110]  Pabcp=[10e3 9e3 11e3]  QLabcp=[100 90 110]  QCabcp=[100 90 110]  Measurements=None  LoadType=constant Z
  MAN7 : spsThreePhaseVIMeasurementLib/Three-Phase V-I Measurement  VoltageMeasurement=no  SetLabelV=on  LabelV=Vabc_MAN7  Vpu=on  VpuLL=off  CurrentMeasurement=no  SetLabelI=on  LabelI=Iabc_MAN7  Ipu=on  Pbase=100e6  Vbase=735e3  OutputType=Magnitude  PhasorSimulation=off  PSBequivalent=0
  MIC-LTD 409 km : spsDistributedParametersLineLib/Distributed Parameters Line  Phases=3  Length=409  Frequency=60  Resistance="[0.01273  0.3864]"  Inductance="[0.9337e-3  4.1264e-3]"  Capacitance=[12.74e-9 7.751e-9]  x1=[-0.002325 4.67266995586132e-09 0 0;-0.00225 4.68287077338809e-09 0 0;-0.002175 4.68932817566895e-09 0 0;-0.0021 4.69203700075529e-09 0 0;-0.002025 4.69099508325381e-09 0 0;-0.00195 4.68620325605741e-09 0 0;-0.001875 4.67766534967943e-09 0 0;-0.0018 4.6653881891916e-09 0 0;-0.001725 4.64938158876815e-09 0 0;-0.00165 4.62965834384058e-09 0 0;-0.001575 4.60623422086908e-09 0 0;-0.0015 4.57912794473917e-09 0 0;-0.001425 4.54836118379324e-09 59193.0163102594 -807702.943453792;-0.00135 4.51395853250924e-09 82003.6023342162 -805706.722468983;-0.001275 4.47594749184024e-09 104748.635933164 -803066.431857958;-0.0012 4.43435844723056e-09 127409.935075255 -799784.182228635;-0.001125 4.38922464432612e-09 149969.384664684 -795862.597361146;-0.00105 4.34058216239839e-09 172408.951022621 -791304.812110433;-0.000975 4.28846988550317e-09 194710.696303056 -786114.469900289;-0.0009 4.23292947139728e-09 216856.792832039 -780295.719810861;-0.000825 4.17400531823794e-09 238829.537358853 -773853.213261941;-0.00075 4.11174452909163e-09 260611.365207717 -766792.100294691;-0.000675 4.04619687428056e-09 282184.864318721 -759118.025454777;-0.0006 3.97741475159708e-09 303532.789166762 -750837.123280211;-0.000525 3.90545314441765e-09 324638.07454735 -741956.013397487;-0.00045 3.83036957775002e-09 345483.849218275 -732481.795229961;-0.000375 3.75222407224856e-09 366053.449386214 -722422.042322676;-0.0003 3.67107909623469e-09 386330.43202752 -711784.796288186;-0.000225 3.58699951576069e-09 406298.588032517 -700578.560378215;-0.00015 3.50005254275672e-09 425941.955162817 -688812.29268629;-7.5e-05 3.41030768130267e-09 445244.830811291 -676495.398986773]  x2=[-0.002325 1.40059135918308e-08 0 0;-0.00225 1.40946192787261e-08 0 0;-0.002175 1.41720579426248e-08 0 0;-0.0021 1.4238167680244e-08 0 0;-0.002025 1.42928956444709e-08 0 0;-0.00195 1.43361980866081e-08 0 0;-0.001875 1.43680403913462e-08 0 0;-0.0018 1.43883971044338e-08 0 0;-0.001725 1.4397251953026e-08 0 0;-0.00165 1.43945978586922e-08 0 0;-0.001575 1.4380436943075e-08 0 0;-0.0015 1.43547805261935e-08 0 0;-0.001425 1.43176491173949e-08 -248116.944399225 -772658.724453944;-0.00135 1.42690723989592e-08 -226174.261593797 -779364.307396023;-0.001275 1.4209089202372e-08 -204050.778544234 -785446.878435444;-0.0012 1.41377474772827e-08 -181764.180424385 -790901.575257983;-0.001125 1.40551042531748e-08 -159332.282799789 -795724.037462462;-0.00105 1.39612255937773e-08 -136773.017386189 -799910.410046378;-0.000975 1.3856186544254e-08 -114104.417715188 -803457.346487544;-0.0009 1.3740071071214e-08 -91344.604718521 -806362.011419237;-0.000825 1.36129719955899e-08 -68511.7722424616 -808622.082896754;-0.00075 1.34749909184379e-08 -45624.1725039369 -810235.754253535;-0.000675 1.33262381397199e-08 -22700.1014999858 -811201.73554539;-0.0006 1.31668325701314e-08 242.115617781237 -811519.254581652;-0.000525 1.29969016360456e-08 23184.1391920279 -811188.057542463;-0.00045 1.28165811776512e-08 46107.6297201337 -810208.409181668;-0.000375 1.26260153403637e-08 68994.2625145116 -808581.092615177;-0.0003 1.24253564595976e-08 91825.742351083 -806307.408694955;-0.000225 1.2214764938992e-08 114583.8180942 -803389.17496914;-0.00015 1.19944091221863e-08 137250.297286324 -799828.72422912;-7.5e-05 1.1764465158249e-08 159807.060690796 -795628.902644742]  x3=[-0.002325 3.18763869599653e-12 0 0;-0.00225 3.7023499053296e-12 0 0;-0.002175 4.21410151279621e-12 0 0;-0.0021 4.72248443199139e-12 0 0;-0.002025 5.22709226938809e-12 0 0;-0.00195 5.72752164920182e-12 0 0;-0.001875 6.22337253584321e-12 0 0;-0.0018 6.71424855370023e-12 0 0;-0.001725 7.19975730399487e-12 0 0;-0.00165 7.67951067846068e-12 0 0;-0.001575 8.15312516959059e-12 0 0;-0.0015 8.62022217720691e-12 0 0;-0.001425 9.08042831110861e-12 -412.085781584367 -775.710829515009;-0.00135 9.53337568955362e-12 -389.991383899432 -787.050857738252;-0.001275 9.97870223333793e-12 -367.585233069277 -797.7617295481;-0.0012 1.04160519552362e-11 -344.885240228048 -807.834882837511;-0.001125 1.08450752445724e-11 -321.909551402703 -817.262265281871;-0.00105 1.12654291466932e-11 -298.676533007347 -826.036340775896;-0.000975 1.16767776371211e-11 -275.204757161409 -834.150095457884;-0.0009 1.20787918901665e-11 -251.512986843371 -841.597043316488;-0.000825 1.24711505417867e-11 -227.620160891927 -848.371231375532;-0.00075 1.28535399464787e-11 -203.545378866572 -854.467244452729;-0.000675 1.32256544280033e-11 -179.3078857797 -859.880209488497;-0.0006 1.35871965237374e-11 -154.927056712438 -864.605799441409;-0.000525 1.39378772224616e-11 -130.422381326504 -868.64023674716;-0.00045 1.42774161953907e-11 -105.813448284466 -871.980296338296;-0.000375 1.46055420202651e-11 -81.1199295908705 -874.623308222286;-0.0003 1.49219923983208e-11 -56.3615648667361 -876.567159615868;-0.000225 1.52265143639674e-11 -31.5581455700082 -877.81029663398;-0.00015 1.55188644870049e-11 -6.72949917456732 -878.351725531911;-7.5e-05 1.57988090672181e-11 18.1045266795489 -878.191013499684]  x4=[-0.002325 1.58311578884584e-11 0 0;-0.00225 1.57223833373677e-11 0 0;-0.002175 1.56010405535976e-11 0 0;-0.0021 1.5467226536713e-11 0 0;-0.002025 1.53210482555914e-11 0 0;-0.00195 1.51626225629141e-11 0 0;-0.001875 1.4992076101756e-11 0 0;-0.0018 1.48095452043486e-11 0 0;-0.001725 1.46151757830985e-11 0 0;-0.00165 1.4409123213947e-11 0 0;-0.001575 1.41915522121653e-11 0 0;-0.0015 1.39626367006832e-11 0 0;-0.001425 1.37225596710581e-11 -1850.18013712952 -4788.0957463622;-0.00135 1.34715130371942e-11 -1714.07818949526 -4838.48753312458;-0.001275 1.32096974819294e-11 -1576.60603398259 -4885.01150698432;-0.0012 1.29373222966127e-11 -1437.87356372924 -4927.63047738856;-0.001125 1.26546052137997e-11 -1297.99167934924 -4966.31037538445;-0.00105 1.23617722332008e-11 -1157.07220028071 -5001.02028085335;-0.000975 1.20590574410201e-11 -1015.22777539908 -5031.73244722792;-0.0009 1.17467028228309e-11 -872.571792967296 -5058.42232367226;-0.000825 1.14249580701356e-11 -729.218289995011 -5081.06857470751;-0.00075 1.10940803807668e-11 -585.281861079119 -5099.6530972671;-0.000675 1.07543342532867e-11 -440.877566798592 -5114.16103516805;-0.0006 1.04059912755514e-11 -296.12084173682 -5124.58079098676;-0.000525 1.00493299076075e-11 -151.127402204965 -5130.90403532988;-0.00045 9.68463525909524e-12 -6.01315374011278 -5133.12571349262;-0.000375 9.31219886133679e-12 139.105901547834 -5131.24404949945;-0.0003 8.93231843429001e-12 284.113757706476 -5125.26054752378;-0.000225 8.54529764855591e-12 428.894497674293 -5115.17999068553;-0.00015 8.151445882629e-12 573.332385942976 -5101.01043722761;-7.5e-05 7.75107797558482e-12 717.311961074615 -5082.76321407424]  x5=0.00231306500901259  V1=ones(3,3)  V2=ones(3,3)  I1=ones(3,3)  I2=ones(3,3)  nHarmo=1  Measurements=None  Decoupling=on  VsMag0=[661255.450009721 661256.198077798 661255.233015218]  VrMag0=[662602.894278608 662603.037872478 662602.726163221]  VsAngle0=[4.97147028275105 -115.028588850413 124.971384582246]  VrAngle0=[-17.0228975012821 -137.022921456009 102.977079768198]  IsMag0=[724.117205145546 724.119993409772 724.122226064432]  IrMag0=[4231.68630935715 4231.68661611251 4231.68036878049]  IsAngle0=[-27.1991957967951 -147.198864433654 92.8007788226558]  IrAngle0=[-20.3470720252917 -140.347167299997 99.6528767404197]
      settings: AttributesFormatString=\n  LibrarySourceBlock=sps_lib/Power Grid Elements/Distributed Parameters Line
  MIC-MAN 60 km : spsDistributedParametersLineLib/Distributed Parameters Line  Phases=3  Length=60  Frequency=60  Resistance="[0.01273  0.3864]"  Inductance="[0.9337e-3  4.1264e-3]"  Capacitance=[12.74e-9 7.751e-9]  x1=[-0.000375 3.95381031530078e-09 327054.20533703 -753828.913938379;-0.0003 3.86757833860152e-09 348234.666111794 -744281.641234026;-0.000225 3.77825467895431e-09 369136.753422638 -734139.401173561;-0.00015 3.68591074032598e-09 389743.758460777 -723410.301308507;-7.5e-05 3.59062034104816e-09 410039.208301682 -712102.918317136]  x2=[-0.000375 1.07742798642558e-09 341757.375055633 -724337.843086576;-0.0003 1.02648156742245e-09 362098.228966637 -714386.690108679;-0.000225 9.7471459476002e-10 382149.627093695 -703864.467341192;-0.00015 9.2216845016417e-10 401895.540655938 -692779.586088001;-7.5e-05 8.68885138218909e-10 421320.18507219 -681140.907433573]  x3=[-0.000375 -1.5520641678043e-11 2516.12263919172 -3470.38246360564;-0.0003 -1.62031463117031e-11 2613.22665570717 -3397.86332962454;-0.000225 -1.68726983981181e-11 2708.24169881776 -3322.6279956868;-0.00015 -1.75287627075946e-11 2801.09181495179 -3244.73660376722;-7.5e-05 -1.81708147923617e-11 2891.7027811471 -3164.25141905272]  x4=[-0.000375 2.17809637523961e-11 -263.637973265597 -2074.49907539859;-0.0003 2.23848564809202e-11 -204.885257542301 -2081.1231946389;-0.000225 2.29708550976733e-11 -145.968759678976 -2086.08369583967;-0.00015 2.35384911643271e-11 -86.9355766225599 -2089.37661365214;-7.5e-05 2.40873109212952e-11 -27.8328985963508 -2090.99931576818]  x5=0.000339324940197445  V1=ones(3,3)  V2=ones(3,3)  I1=ones(3,3)  I2=ones(3,3)  nHarmo=1  Measurements=None  Decoupling=on  VsMag0=[670930.718084371 670931.402748966 670930.538861449]  VrMag0=[653943.402704874 653944.061381525 653943.21471976]  VsAngle0=[1.55396261636306 -118.446088813405 121.553886266144]  VrAngle0=[3.35889302260881 -116.641159315006 123.358816875026]  IsMag0=[3504.88423853023 3504.88739130355 3504.88350496874]  IrMag0=[1709.85567574013 1709.8580489713 1709.85543949948]  IsAngle0=[14.0431472467737 -105.956896356642 134.043080810377]  IrAngle0=[-29.1426028746229 -149.142657929221 90.8573007274505]
      settings: AttributesFormatString=\n  LibrarySourceBlock=sps_lib/Power Grid Elements/Distributed Parameters Line
  Regulateurs6 : Subsystem
  Regulateurs7 : Subsystem
  "MIC7a " : PMIOPort  Side=Left
  MIC7b : PMIOPort  Port=2  Side=Left
  MIC7c : PMIOPort  Port=3  Side=Left
  QUE7a : PMIOPort  Port=4  Side=Left
  QUE7b : PMIOPort  Port=5  Side=Left
  QUE7c : PMIOPort  Port=6  Side=Left
  wires:
  Regulateurs6/1(Pm) -> "B_6 CHU-5600 MVA "/1
  Regulateurs6/2(Vf) -> "B_6 CHU-5600 MVA "/2
  "B_6 CHU-5600 MVA "/1 -> Regulateurs6/1(m)
  Regulateurs7/1(Pm) -> B_7 MAN 5000 MVA/1
  Regulateurs7/2(Vf) -> B_7 MAN 5000 MVA/2
  B_7 MAN 5000 MVA/1 -> Regulateurs7/1(m)
  connections:
  "Cs PER "/RConn3 -- MIC-LTD 409 km/LConn3
  "Cs PER "/RConn2 -- MIC-LTD 409 km/LConn2
  "Cs PER "/RConn1 -- MIC-LTD 409 km/LConn1
  Cs BER/RConn3 -- MAN-LEV 3*379km/LConn3
  Cs BER/RConn2 -- MAN-LEV 3*379km/LConn2
  Cs BER/RConn1 -- MAN-LEV 3*379km/LConn1
  Cs ARNS2/RConn3 -- ARN-MAN 2*169km/LConn3
  Cs ARNS2/RConn2 -- ARN-MAN 2*169km/LConn2
  Cs ARNS2/RConn1 -- ARN-MAN 2*169km/LConn1
  CHU-ARN 3*450km/RConn3 -- "Cs MTG+ARNN "/LConn3
  CHU-ARN 3*450km/RConn2 -- "Cs MTG+ARNN "/LConn2
  CHU-ARN 3*450km/RConn1 -- "Cs MTG+ARNN "/LConn1
  Load Flow Bus2/LConn1 -- 5600 MVA 13.8 kV/735 kV1/RConn3 -- CHU-ARN 3*450km/LConn3 -- CHU 330 Mvar/LConn3
  5600 MVA 13.8 kV/735 kV1/RConn2 -- CHU-ARN 3*450km/LConn2 -- CHU 330 Mvar/LConn2
  5600 MVA 13.8 kV/735 kV1/RConn1 -- CHU-ARN 3*450km/LConn1 -- CHU 330 Mvar/LConn1
  "B_6 CHU-5600 MVA "/RConn3 -- Load Flow Bus1/LConn1 -- 5600 MVA 13.8 kV/735 kV1/LConn3 -- 280 MW/LConn3
  5600 MVA 13.8 kV/735 kV1/LConn2 -- "B_6 CHU-5600 MVA "/RConn2 -- 280 MW/LConn2
  5600 MVA 13.8 kV/735 kV1/LConn1 -- "B_6 CHU-5600 MVA "/RConn1 -- 280 MW/LConn1
  "Cs ARNS1 "/RConn1 -- ARN-MIC 180km/LConn1
  "Cs ARNS1 "/RConn2 -- ARN-MIC 180km/LConn2
  "Cs ARNS1 "/RConn3 -- ARN-MIC 180km/LConn3
  "Cs PER "/LConn3 -- Load Flow Bus6/LConn1 -- MIC7c/RConn1 -- MIC-MAN 60 km/LConn3 -- ARN-MIC 180km/RConn3
  "Cs PER "/LConn2 -- MIC7b/RConn1 -- ARN-MIC 180km/RConn2 -- MIC-MAN 60 km/LConn2
  "Cs PER "/LConn1 -- "MIC7a "/RConn1 -- ARN-MIC 180km/RConn1 -- MIC-MAN 60 km/LConn1
  ARN-MAN 2*169km/RConn1 -- MAN7/LConn1
  ARN-MAN 2*169km/RConn2 -- MAN7/LConn2
  ARN-MAN 2*169km/RConn3 -- MAN7/LConn3
  Cs BER/LConn1 -- 5000 MVA 13.8 kV/735 kV2/RConn1 -- MIC-MAN 60 km/RConn1 -- MAN-MIC 1650 Mvar/LConn1 -- MAN7/RConn1
  Cs BER/LConn2 -- 5000 MVA 13.8 kV/735 kV2/RConn2 -- MIC-MAN 60 km/RConn2 -- MAN-MIC 1650 Mvar/LConn2 -- MAN7/RConn2
  Cs BER/LConn3 -- Load Flow Bus5/LConn1 -- 5000 MVA 13.8 kV/735 kV2/RConn3 -- MIC-MAN 60 km/RConn3 -- MAN-MIC 1650 Mvar/LConn3 -- MAN7/RConn3
  B_7 MAN 5000 MVA/RConn1 -- 5000 MVA 13.8 kV/735 kV2/LConn1 -- 250 MW/LConn1
  B_7 MAN 5000 MVA/RConn2 -- 5000 MVA 13.8 kV/735 kV2/LConn2 -- 250 MW/LConn2
  B_7 MAN 5000 MVA/RConn3 -- 5000 MVA 13.8 kV/735 kV2/LConn3 -- Load Flow Bus3/LConn1 -- 250 MW/LConn3
  MIC-LTD 409 km/RConn2 -- MAN-LEV 3*379km/RConn2 -- QUE7b/RConn1
  Cs ARNS2/LConn1 -- ARN 990 Mvar/LConn1 -- "Cs MTG+ARNN "/RConn1 -- "Cs ARNS1 "/LConn1
  Cs ARNS2/LConn2 -- ARN 990 Mvar/LConn2 -- "Cs MTG+ARNN "/RConn2 -- "Cs ARNS1 "/LConn2
  Cs ARNS2/LConn3 -- Load Flow Bus4/LConn1 -- "Cs ARNS1 "/LConn3 -- ARN 990 Mvar/LConn3 -- "Cs MTG+ARNN "/RConn3
  MIC-LTD 409 km/RConn1 -- QUE7a/RConn1 -- MAN-LEV 3*379km/RConn1
  MIC-LTD 409 km/RConn3 -- QUE7c/RConn1 -- MAN-LEV 3*379km/RConn3
